simulink model "ansiOct"  (R2018a)
settings: Solver=VariableStepAuto  StartTime=0.0  StopTime=0.1  RelTol=1e-3
undefined symbols (not defined in the file or in its folder): fdesignblkfcn, G1, G2, G3, G4, G5, G6, G7, G8, gcbh, get, T
libraries: dspsrcs4 x1, dspxfrm3 x1, dspobslib x1
(part 2 of 4)

== system ansiOct/Filter Bank /Filter 2/Bandpass Filter ==
  In : Inport
  Generated Filter Block : DiscreteFir  Tag=BlockMethodSubSystem  Coefficients=[-0.00683808473801020538 0.000453146012099650791 0.000439193334597743983 0.000425688735826898403 0.000413372222263871545 0.00040142288334680062 0.00039058929220634847 0.00038004506436549782 0.000370562120820603529 0.000361285945627898774 0.000353023210082561154 0.000344891623023386355 0.000337733977270703381 0.000330627325545598729 0.000324469668998443855 0.00031828100727470792 0.000313026450039366173 0.00030765203845560887 0.000303212557918509538 0.000298555264758741342 0.000294854525948781753 0.000290821386413294347 0.000287795197852407612 0.000284291020882040718 0.000281885977117910837 0.000278810014255677688 0.000277002847052887184 0.000274222537854552472 0.000273046170456389659 0.000270339423992273177 0.000270019954982382755 0.000266445025573808453 0.000273046934952013421 0.000257459599699634654 0.000261462285937973614 0.000266910849645362344 0.000265585248307291272 0.000264843364974099349 0.000261914436451702172 0.000260645770105994757 0.000258697261520209683 0.000258379723815770437 0.000257602576687380091 0.000258013220566671397 0.000257822365293245792 0.000258405835838067125 0.000258247613458107198 0.000258614819179062367 0.000258202625373678968 0.000258221855966103274 0.000257500697546511625 0.000257215456059062297 0.000256259089873529138 0.000255790355165799212 0.000254705424987607858 0.000254173874873210993 0.000253038508008838797 0.000252522278059655195 0.000251354195672259014 0.000250897784056915726 0.000249647530087847942 0.000249281000714943418 0.000247805266176076707 0.000247724874810998329 0.000245043919941419718 0.000247004073907041994 0.000243712518480117225 0.000241006312647941488 0.000241662134215342905 0.000240502346996609637 0.000239248910919219189 0.000236746646484521758 0.000234632998992699679 0.000232152226948542461 0.000230229089791924392 0.000228035323948653839 0.000226129735824407064 0.000223790088876914072 0.000221520436286805518 0.00021876675472485321 0.000216054507524204197 0.00021294240861747816 0.000209950984414387931 0.000206664790313006863 0.000203571595373398985 0.000200232009745841941 0.000197110704457774844 0.00019372303616359347 0.000190544567683604914 0.000187038924090264589 0.000183735590096929005 0.000180021416210796883 0.000176554224089025158 0.000172569132625265473 0.000168963532991142542 0.000164624753670193326 0.000161155770817601084 0.000156031342534981279 0.000152672428214057168 0.000148791175363421137 0.000143068185378687681 0.000139189114071677707 0.000134984310436230643 0.000130964714553581576 0.000126161826510100148 0.000121496872691168899 0.000116548934979699643 0.000111974843739821685 0.000107256327152767134 0.000102766188905174271 9.79952193671045725e-05 9.32944181421482577e-05 8.82818880088702846e-05 8.33510504216724885e-05 7.82012213752934278e-05 7.32204012976075236e-05 6.81070951341132373e-05 6.32065348646243156e-05 5.81853745438533289e-05 5.33681833614937213e-05 4.83983302302114281e-05 4.36159689608017266e-05 3.86515001921420388e-05 3.38940204356166907e-05 2.89322900133945522e-05 2.42453661543740962e-05 1.93242467940092468e-05 1.48002666285436156e-05 9.89089137550368071e-06 5.71416651658179511e-06 8.69847030465080218e-07 -3.6814496531191979e-06 -7.22035679483634182e-06 -1.21369059114201459e-05 -1.64244060690918079e-05 -2.05468988703493851e-05 -2.43066795068125194e-05 -2.83563901396811314e-05 -3.23577189466347378e-05 -3.64674813471225695e-05 -4.03068446993442745e-05 -4.40567305726795143e-05 -4.75443860945283145e-05 -5.10191973534812344e-05 -5.43467812918436443e-05 -5.76999438030773216e-05 -6.08973829637311919e-05 -6.40545427075864515e-05 -6.69901713590295261e-05 -6.9832813742601058e-05 -7.24403759680233606e-05 -7.49762890148145307e-05 -7.73120258976689321e-05 -7.9617814251851471e-05 -8.17448391247448363e-05 -8.38582457624153648e-05 -8.57653295073239086e-05 -8.76560959961967661e-05 -8.92868054801280433e-05 -9.09082807756561475e-05 -9.21873933758695204e-05 -9.35555707488250002e-05 -9.45020327101644627e-05 -9.53128423085423845e-05 -9.65645109480432398e-05 ...(+41516 chars)]  InputProcessing=Columns as channels (frame based)
  Out : Outport
  wires:
  In/1 -> Generated Filter Block/1
  Generated Filter Block/1 -> Out/1
